simulink model "rs_latch"  (R2024a)
settings: Solver=FixedStepDiscrete  StartTime=1  StopTime=inf  RelTol=1e-3  EnableMultiTasking=on
settings Model: Creator=nunkesser  LastModifiedBy=nunkesser
settings SolverCC: AlgebraicLoopSolver=TrustRegion
settings DataIOCC: LimitDataPoints=on  SaveFormat=Array  ReturnWorkspaceOutputs=off
settings OptimizationCC: LifeSpan=inf
settings DebuggingCC: SolverPrmCheckMsg=warning  UnconnectedInputMsg=warning  UnconnectedOutputMsg=warning  UnconnectedLineMsg=warning  SFUnexpectedBacktrackingDiag=warning  SFNoUnconditionalDefaultTransitionDiag=warning  SFExecutionAtInitializationDiag=none  ArithmeticOperatorsInVariantConditions=warning
settings HardwareCC: ProdBitPerPointer=32  ProdBitPerSizeT=32  ProdBitPerPtrDiffT=32  ProdLargestAtomicFloat=None  ProdIntDivRoundTo=Undefined  ProdEndianess=Unspecified  ProdWordSize=32  ProdHWDeviceType=32-bit Generic
settings ModelReferenceCC: PropagateSignalLabelsOutOfModel=off
settings SFSimCC: SimUseLocalCustomCode=off  CustomCodeUndefinedFunction=UseInterfaceOnly
settings RTWCC: RTWUseLocalCustomCode=off  GPUComputeCapability=3.5
settings CodeAppCC: StateflowObjectComments=on
settings GRTTargetCC: TargetLangStandard=C89/C90 (ANSI)
settings ConfigComp: CovMetricSettings=dw  CovSaveCumulativeToWorkspaceVar=on  CovSaveSingleToWorkspaceVar=on  CovExternalEMLEnable=off  CovSFcnEnable=off
settings ConfigurationSet: Description=SimMechanics 2G

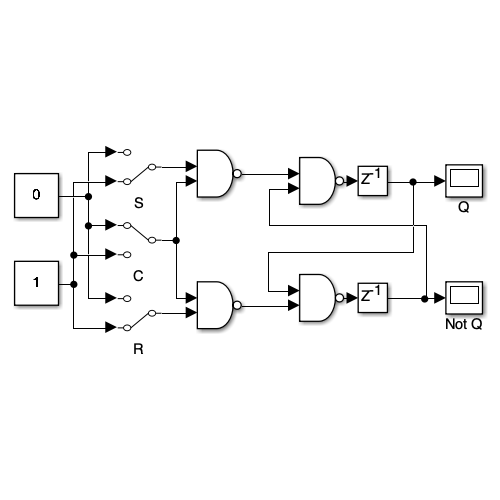
[thumbnail: Simulink's stored preview of the top-level diagram]
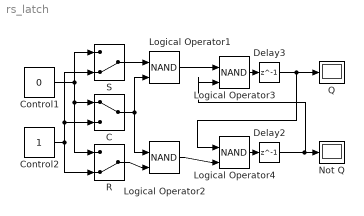
== system rs_latch ==
  C : ManualSwitch
  Control1 : Constant  Value=0  OutDataTypeStr=boolean
  Control2 : Constant  OutDataTypeStr=boolean
  Delay2 : Delay  DelayLength=1  InitialCondition=0
  Delay3 : Delay  DelayLength=1  InitialCondition=0
  Logical Operator{1..4} (4 alike) : Logic  Operator=NAND  IconShape=distinctive  AllPortsSameDT=off  OutDataTypeStr=boolean
  Not Q : Display
  Q : Display
  R : ManualSwitch  CurrentSetting=0
  S : ManualSwitch  CurrentSetting=0
  wires:
  Logical Operator3/1 -> Delay3/1
  S/1 -> Logical Operator1/1
  C/1 -> Logical Operator1/2, Logical Operator2/1
  R/1 -> Logical Operator2/2
  Control1/1 -> R/1, C/1, S/1
  Control2/1 -> R/2, S/2, C/2
  Logical Operator4/1 -> Delay2/1
  Delay2/1 -> Not Q/1, Logical Operator3/2
  Delay3/1 -> Q/1, Logical Operator4/1
  Logical Operator2/1 -> Logical Operator4/2
  Logical Operator1/1 -> Logical Operator3/1
